simulink model "Mars_escape_sim"  (R2024b)
settings: Solver=VariableStepAuto  StartTime=0.0  StopTime=5e5  MaxStep=50  RelTol=1e-6
values from neighbouring files (symbols this model uses):
  mars_escape_data = escape(Mars_planet,orbit_data,transfer_inbound_data,escape_burn_time)    [Mars_escape_setup.m]
  transfer_inbound_data = hohmann_transfer(Mars_inbound,Earth_inbound,Sun_mu,burn_time)    [Hohmann_setup.m]
settings Model: Creator=cpero  LastModifiedBy=cpero

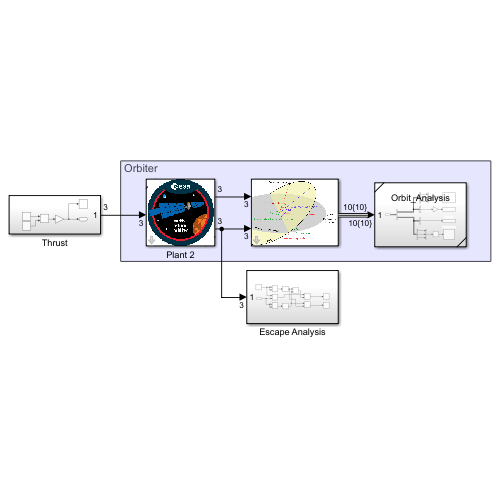
[thumbnail: Simulink's stored preview of the top-level diagram]
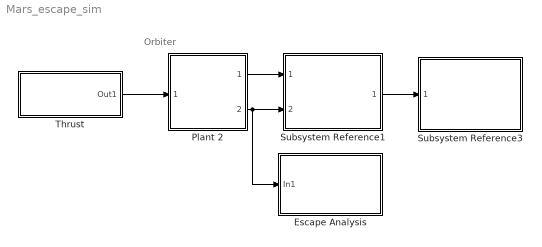
== system Mars_escape_sim ==
  note: Orbiter
  Escape Analysis : Subsystem
  Plant 2 : Subsystem  ReferencedSubsystem=Plant  setup=mars_escape_data.orbiter_initial  switch_time=0  mu=Mars_planet.mu
  Subsystem Reference1 : Subsystem  ReferencedSubsystem=Orbit_Calculations  mu=Mars_planet.mu
  Subsystem Reference3 : Subsystem  ReferencedSubsystem=Orbit_Analysis
  Thrust : Subsystem
  wires:
  Plant 2/1 -> Subsystem Reference1/1
  Subsystem Reference1/1 -> Subsystem Reference3/1
  Thrust/1(Out1) -> Plant 2/1
  Plant 2/2 -> Escape Analysis/1(In1), Subsystem Reference1/2

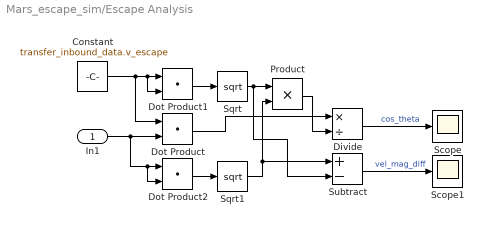
== system Mars_escape_sim/Escape Analysis ==
  In1 : Inport
  Constant : Constant  Value=transfer_inbound_data.v_escape
  Divide : Product  Inputs=*/
  Dot Product : DotProduct  OutDataTypeStr=Inherit: Inherit via internal rule
  Dot Product1 : DotProduct  OutDataTypeStr=Inherit: Inherit via internal rule
  Dot Product2 : DotProduct  OutDataTypeStr=Inherit: Inherit via internal rule
  Product : Product
  Scope : Scope
  Scope1 : Scope
  Sqrt : Sqrt
  Sqrt1 : Sqrt
  Subtract : Sum  Inputs=+-
  wires:
  Constant/1 -> Dot Product1/2, Dot Product1/1, Dot Product/1
  Dot Product1/1 -> Sqrt/1
  Dot Product2/1 -> Sqrt1/1
  In1/1 -> Dot Product2/2, Dot Product2/1, Dot Product/2
  Sqrt/1 -> Subtract/2, Product/1
  Sqrt1/1 -> Product/2, Subtract/1
  Divide/1 -> Scope/1  "cos_theta"
  Product/1 -> Divide/2
  Dot Product/1 -> Divide/1
  Subtract/1 -> Scope1/1  "vel_mag_diff"

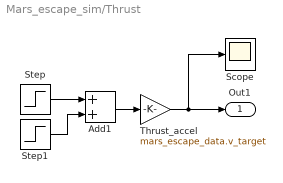
== system Mars_escape_sim/Thrust ==
  Add1 : Sum
  Scope : Scope
  Step : Step  Time=mars_escape_data.time  SampleTime=0
  Step1 : Step  Time=mars_escape_data.time + 1  After=-1  SampleTime=0
  Thrust_accel : Gain  Gain=mars_escape_data.v_target
  Out1 : Outport
  wires:
  Add1/1 -> Thrust_accel/1
  Thrust_accel/1 -> Out1/1, Scope/1
  Step1/1 -> Add1/2
  Step/1 -> Add1/1
